simulink model "Simple_4Quad_payload_09_2017a"  (R2018b)
settings: Solver=ode45  StartTime=0.0  StopTime=40  RelTol=1e-3
InitFcn:
  | Simple_4Quad_payload_09_const
values from neighbouring files (symbols this model uses):
  All_rho = [d1 0 0 ... (first row only)    [Colab_4Quad_model_01_const.m]    (also in Colab_4Quad_model_02_const.m; Simple_4Quad_payload_04_const.m; Simple_4Quad_payload_05_const.m; Simple_4Quad_payload_06_const.m)
  alpha_chatt = 0.1    [Simple_4Quad_payload_09_const.m]    (also in Simple_4Quad_payload_10_const.m = 0.001; Simple_4Quad_payload_11_const.m = 0.01; Simple_4Quad_payload_12_const.m = 0.01)
  alphaTF = 0.1    [Simple_4Quad_payload_08_const.m]    (also in Simple_4Quad_payload_09_const.m = 0.5; Simple_4Quad_payload_10_const.m = 1; Simple_4Quad_payload_11_const.m = 0.5; Simple_4Quad_payload_12_const.m = 10)
  B_ob = [zeros(3);eye(3)]    [Simple_4Quad_payload_04_const.m]    (also in Simple_4Quad_payload_05_const.m; Simple_4Quad_payload_06_const.m; Simple_4Quad_payload_07_const.m; Simple_4Quad_payload_08_const.m)
  BBT_inv = ((B'*B)^(-1))*B'    [Simple_2Quad_payload_03_const.m]    (also in Simple_4Quad_payload_04_const.m = ((BR'*BR)^(-1))*BR'; Simple_4Quad_payload_05_const.m = ((BR'*BR)^(-1))*BR'; Simple_4Quad_payload_06_const.m = ((BR'*BR)^(-1))*BR'; Simple_4Quad_payload_07_const.m = ((BR'*BR)^(-1))*BR')
  BR = 1e0*eye(n)    [Simple_4Quad_payload_04_const.m]    (also in Simple_4Quad_payload_05_const.m; Simple_4Quad_payload_06_const.m; Simple_4Quad_payload_07_const.m; Simple_4Quad_payload_08_const.m)
  C_ob = [eye(3) zeros(3)]    [Simple_4Quad_payload_04_const.m]    (also in Simple_4Quad_payload_05_const.m; Simple_4Quad_payload_06_const.m; Simple_4Quad_payload_07_const.m; Simple_4Quad_payload_08_const.m)
  d1 = 0.25    [Colab_4Quad_model_01_const.m]    (also in Colab_4Quad_model_02_const.m = 0.5; Simple_4Quad_payload_01_const.m = 1; Simple_4Quad_payload_02_const.m = 1; Simple_4Quad_payload_03_const.m = 1)
  d2 = 0.25    [Colab_4Quad_model_01_const.m]    (also in Colab_4Quad_model_02_const.m = 0.5; Simple_4Quad_payload_01_const.m = 1; Simple_4Quad_payload_02_const.m = 1; Simple_4Quad_payload_03_const.m = 1)
  Des_rel_dist = 2    [Simple_4Quad_payload_01_const.m]    (also in Simple_4Quad_payload_02_const.m = 4; Simple_4Quad_payload_03_const.m = 4; Simple_4Quad_payload_04_const.m; Simple_4Quad_payload_05_const.m)
  g = 9.81    [Colab_4Quad_model_01_const.m]    (also in Colab_4Quad_model_02_const.m; Simple_2Quad_payload_01_const.m; Simple_2Quad_payload_02_const.m; Simple_2Quad_payload_03_const.m)
  gamma_0 = 1e-0*diag([1e-3;1e-0])    [Simple_2Quad_payload_03_const.m]    (also in Simple_4Quad_payload_04_const.m = 1e-0*diag([1e-6*ones(3,1);1e-0*ones(3,1)]); Simple_4Quad_payload_05_const.m = 1e-1*diag([1e-6*ones(3,1);1e-0*ones(3,1)]); Simple_4Quad_payload_06_const.m = 1e-0*diag([1e-6*ones(3,1);1e-0*ones(3,1)]); Simple_4Quad_payload_07_const.m = 1e-0*diag([1e-6*ones(3,1);1e-0*ones(3,1)]))
  gamma_0L = 1e-0*diag([1e-6*ones(3,1);1e-0*ones(3,1)])    [Simple_4Quad_payload_08_const.m]    (also in Simple_4Quad_payload_09_const.m; Simple_4Quad_payload_10_const.m = 1e+0*diag([1e-3*ones(3,1);1e-3*ones(3,1)]); Simple_4Quad_payload_11_const.m = 1e+0*diag([1e-3*ones(3,1);1e-3*ones(3,1)]); Simple_4Quad_payload_12_const.m = 1e+2*diag(1e-4*ones(3,1)))
  gamma_0v = 1e-0*diag([1e-0*ones(3,1);1e-0*ones(3,1)])    [Simple_4Quad_payload_08_const.m]    (also in Simple_4Quad_payload_09_const.m = 1e-0*diag([1e-6*ones(3,1);1e-6*ones(3,1)]); Simple_4Quad_payload_10_const.m = 1e+0*diag(1e-0*ones(3,1)); Simple_4Quad_payload_11_const.m = 1e+0*diag(1e-0*ones(3,1)); Simple_4Quad_payload_12_const.m = 1e+3*diag(1e-0*ones(3,1)))
  gamma_1 = 1e+2*diag([1e-3;1e-0])    [Simple_2Quad_payload_03_const.m]    (also in Simple_4Quad_payload_04_const.m = 1e+2*diag([1e-6*ones(3,1);1e-0*ones(3,1)]); Simple_4Quad_payload_05_const.m = 1e+2*diag([1e-6*ones(3,1);1e-0*ones(3,1)]); Simple_4Quad_payload_06_const.m = 1e+3*diag([1e-6*ones(3,1);1e-0*ones(3,1)]); Simple_4Quad_payload_07_const.m = 1e+3*diag([1e-6*ones(3,1);1e-0*ones(3,1)]))
  gamma_1L = 1e+3*diag([1e-6*ones(3,1);1e-0*ones(3,1)])    [Simple_4Quad_payload_08_const.m]    (also in Simple_4Quad_payload_09_const.m = 1e+2*diag([1e-6*ones(3,1);1e-0*ones(3,1)]); Simple_4Quad_payload_10_const.m = 1e+1*diag([1e-3*ones(3,1);1e-3*ones(3,1)]); Simple_4Quad_payload_11_const.m = 1e+0*diag([1e-3*ones(3,1);1e-3*ones(3,1)]); Simple_4Quad_payload_12_const.m = 1e+2*diag(1e-4*ones(3,1)))
  gamma_1v = 1e+3*diag([1e-0*ones(3,1);1e-0*ones(3,1)])    [Simple_4Quad_payload_08_const.m]    (also in Simple_4Quad_payload_09_const.m = 1e+2*diag([1e-6*ones(3,1);1e-6*ones(3,1)]); Simple_4Quad_payload_10_const.m = 1e+0*diag(1e-0*ones(3,1)); Simple_4Quad_payload_11_const.m = 1e+0*diag(1e-0*ones(3,1)); Simple_4Quad_payload_12_const.m = 1e+3*diag(1e-0*ones(3,1)))
  Ix = 0.166667    [Colab_4Quad_model_01_const.m]    (also in Colab_4Quad_model_02_const.m = 0.02; Simple_4Quad_payload_01_const.m = 1; Simple_4Quad_payload_02_const.m = 1; Simple_4Quad_payload_03_const.m = 1)
  Iy = 0.166667    [Colab_4Quad_model_01_const.m]    (also in Colab_4Quad_model_02_const.m = 0.02; Simple_4Quad_payload_01_const.m = 1; Simple_4Quad_payload_02_const.m = 1; Simple_4Quad_payload_03_const.m = 1)
  Iz = 0.166667    [Colab_4Quad_model_01_const.m]    (also in Colab_4Quad_model_02_const.m = 0.02; Simple_4Quad_payload_01_const.m = 1; Simple_4Quad_payload_02_const.m = 1; Simple_4Quad_payload_03_const.m = 1)
  Jo = diag([Ix;Iy;Iz])    [Colab_4Quad_model_01_const.m]    (also in Colab_4Quad_model_02_const.m; Simple_4Quad_payload_04_const.m; Simple_4Quad_payload_05_const.m; Simple_4Quad_payload_06_const.m)
  Jq = diag([0.0291 0.0291 0.0552])    [Colab_4Quad_model_01_const.m]    (also in Colab_4Quad_model_02_const.m = diag([0.03 0.03 0.06]); Simple_4Quad_payload_03_const.m = 1.2416e-3 * diag([1 1 2]); Simple_4Quad_payload_04_const.m = 1 * diag([1 1 2]); Simple_4Quad_payload_05_const.m = 1 * diag([1 1 2]))
  k1 = 1    [Simple_2Quad_payload_03_const.m]    (also in Simple_4Quad_payload_04_const.m; Simple_4Quad_payload_05_const.m; Simple_4Quad_payload_06_const.m; Simple_4Quad_payload_07_const.m)
  k2 = 0.1    [Simple_2Quad_payload_03_const.m]    (also in Simple_4Quad_payload_04_const.m; Simple_4Quad_payload_05_const.m; Simple_4Quad_payload_06_const.m; Simple_4Quad_payload_07_const.m)
  l = 3.1819    [Colab_4Quad_model_01_const.m]    (also in Colab_4Quad_model_02_const.m = 3; Simple_2Quad_payload_04_const.m = 1; Simple_4Quad_payload_01_const.m = 1; Simple_4Quad_payload_02_const.m = 2)
  m = 1.5    [Colab_4Quad_model_01_const.m]    (also in Colab_4Quad_model_02_const.m; Simple_2Quad_payload_04_const.m = 1; Simple_4Quad_payload_01_const.m = 1; Simple_4Quad_payload_02_const.m = 1)
  M = 1.0    (= 1)    [Colab_4Quad_model_01_const.m]    (also in Colab_4Quad_model_02_const.m; Simple_2Quad_payload_01_const.m; Simple_2Quad_payload_02_const.m; Simple_2Quad_payload_03_const.m)
  n = 2    [Simple_2Quad_payload_03_const.m]    (also in Simple_4Quad_payload_03_const.m = 6; Simple_4Quad_payload_04_const.m = 6; Simple_4Quad_payload_05_const.m = 6; Simple_4Quad_payload_06_const.m = 6)
  noise_var_Omegao = 0e-6    (= 0)    [Simple_4Quad_payload_07_const.m]    (also in Simple_4Quad_payload_08_const.m; Simple_4Quad_payload_09_const.m; Simple_4Quad_payload_10_const.m; Simple_4Quad_payload_11_const.m)
  noise_var_RelAcc = 0e-6    (= 0)    [Simple_4Quad_payload_07_const.m]    (also in Simple_4Quad_payload_08_const.m; Simple_4Quad_payload_09_const.m; Simple_4Quad_payload_10_const.m; Simple_4Quad_payload_11_const.m)
  noise_var_RelPos = 0e-6    (= 0)    [Simple_4Quad_payload_07_const.m]    (also in Simple_4Quad_payload_08_const.m; Simple_4Quad_payload_09_const.m; Simple_4Quad_payload_10_const.m; Simple_4Quad_payload_11_const.m)
  Q_ob = var_u_ob * eye(6)    [Simple_4Quad_payload_04_const.m]    (also in Simple_4Quad_payload_05_const.m; Simple_4Quad_payload_06_const.m; Simple_4Quad_payload_07_const.m; Simple_4Quad_payload_08_const.m)
  QL = 1e-0*eye(n)    [Simple_4Quad_payload_08_const.m]    (also in Simple_4Quad_payload_09_const.m; Simple_4Quad_payload_10_const.m; Simple_4Quad_payload_11_const.m = 1e-2*eye(n); Simple_4Quad_payload_12_const.m = 1e-0*eye(np))
  QR = 1e-0*eye(n)    [Simple_4Quad_payload_04_const.m]    (also in Simple_4Quad_payload_05_const.m = 1e-1*eye(n); Simple_4Quad_payload_06_const.m; Simple_4Quad_payload_07_const.m; Simple_4Quad_payload_08_const.m)
  Qv = 1e-0*eye(n)    [Simple_4Quad_payload_08_const.m]    (also in Simple_4Quad_payload_09_const.m; Simple_4Quad_payload_10_const.m = 1e-0*eye(np); Simple_4Quad_payload_11_const.m = 1e-2*eye(np); Simple_4Quad_payload_12_const.m = 1e-0*eye(np))
  R = 1e+0*eye(n)    [Simple_2Quad_payload_03_const.m]    (also in Simple_4Quad_payload_04_const.m = 1e+0*eye(m); Simple_4Quad_payload_05_const.m = 1e+0*eye(m); Simple_4Quad_payload_06_const.m; Simple_4Quad_payload_07_const.m)
  R_ob = var_y_ob * eye(3)    [Simple_4Quad_payload_04_const.m]    (also in Simple_4Quad_payload_05_const.m; Simple_4Quad_payload_06_const.m; Simple_4Quad_payload_07_const.m; Simple_4Quad_payload_08_const.m)
  rho_0 = 1e-0    (= 1)    [Simple_2Quad_payload_03_const.m]    (also in Simple_4Quad_payload_04_const.m; Simple_4Quad_payload_05_const.m = 0.1; Simple_4Quad_payload_06_const.m; Simple_4Quad_payload_07_const.m)
  rho_0L = 1e-0    (= 1)    [Simple_4Quad_payload_08_const.m]    (also in Simple_4Quad_payload_09_const.m; Simple_4Quad_payload_10_const.m; Simple_4Quad_payload_11_const.m; Simple_4Quad_payload_12_const.m)
  rho_0v = 1e-1    (= 0.1)    [Simple_4Quad_payload_08_const.m]    (also in Simple_4Quad_payload_09_const.m = 1; Simple_4Quad_payload_10_const.m = 1; Simple_4Quad_payload_11_const.m = 1; Simple_4Quad_payload_12_const.m = 1)
  rho_1 = 1e-0    (= 1)    [Simple_2Quad_payload_03_const.m]    (also in Simple_4Quad_payload_04_const.m; Simple_4Quad_payload_05_const.m; Simple_4Quad_payload_06_const.m; Simple_4Quad_payload_07_const.m)
  rho_1L = 1e-0    (= 1)    [Simple_4Quad_payload_08_const.m]    (also in Simple_4Quad_payload_09_const.m; Simple_4Quad_payload_10_const.m; Simple_4Quad_payload_11_const.m; Simple_4Quad_payload_12_const.m)
  rho_1v = 1e-0    (= 1)    [Simple_4Quad_payload_08_const.m]    (also in Simple_4Quad_payload_09_const.m; Simple_4Quad_payload_10_const.m; Simple_4Quad_payload_11_const.m; Simple_4Quad_payload_12_const.m)
libraries: simulink x1
(part 4 of 4)

== matlab function Simple_4Quad_payload_09_2017a/Controllers and Observers/Controller and Observer - Agent2/Rotational #2/output definition ==
  data: u input; ur output
function ur = fcn(u)

ur = u(4:6);

end

== matlab function Simple_4Quad_payload_09_2017a/Controllers and Observers/Cotnroller and Observer - Agent1 /Rotational #1/CARE ==
  data: P input; a_hat input; BR parameter; R parameter; DP output; QR parameter
function DP = fcn(P,a_hat,BR,R,QR)

DP = a_hat*P + P*a_hat' - P*BR*R*BR'*P + 2*QR;

end

== matlab function Simple_4Quad_payload_09_2017a/Controllers and Observers/Controlelr and Observer - Agent3/Rotational #3/output definition ==
  data: u input; ur output
function ur = fcn(u)

ur = u(4:6);

end

== matlab function Simple_4Quad_payload_09_2017a/Controllers and Observers/Controller and Observer - Agent4/Rotational #4/output definition ==
  data: u input; ur output
function ur = fcn(u)

ur = u(4:6);

end

== matlab function Simple_4Quad_payload_09_2017a/Dynamic model of the entire system/Control inputs from Q1/Controller Interpreter #1 ==
  data: UTi input; qi input; PHIi input; Ui_local_paral output; PHIo input; Ui_local_perpn output
function [Ui_local_paral,Ui_local_perpn] = fcn(UTi,qi,PHIi,PHIo)

phi_i = PHIi(1);
theta_i = PHIi(2);
psi_i = PHIi(3);

Ri = [cos(psi_i)*cos(theta_i) cos(psi_i)*sin(theta_i)*sin(phi_i)-sin(psi_i)*cos(phi_i) cos(psi_i)*sin(theta_i)*cos(phi_i)+sin(psi_i)*sin(phi_i);
    sin(psi_i)*cos(theta_i) sin(psi_i)*sin(theta_i)*sin(phi_i)+cos(psi_i)*cos(phi_i) sin(psi_i)*sin(theta_i)*cos(phi_i)-cos(psi_i)*sin(phi_i);
    -sin(theta_i) cos(theta_i)*sin(phi_i) cos(theta_i)*cos(phi_i)]; 

phio = PHIo(1);
thetao = PHIo(2);
psio = PHIo(3);

Ro = [cos(psio)*cos(thetao) cos(psio)*sin(thetao)*sin(phio)-sin(psio)*cos(phio) cos(psio)*sin(thetao)*cos(phio)+sin(psio)*sin(phio);
    sin(psio)*cos(thetao) sin(psio)*sin(thetao)*sin(phio)+cos(psio)*cos(phio) sin(psio)*sin(thetao)*cos(phio)-cos(psio)*sin(phio);
    -sin(thetao) cos(thetao)*sin(phio) cos(thetao)*cos(phio)];

Ui_local_paral = (qi*qi') * (eye(3) * Ri * UTi); %Ro'
Ui_local_perpn = (eye(3) - qi*qi') * (eye(3) * Ri * UTi); %Ro'


end

== matlab function Simple_4Quad_payload_09_2017a/Controllers and Observers/Cotnroller and Observer - Agent1 /Link #1/CARE ==
  data: P input; a_hat input; BR parameter; R parameter; DP output; QL parameter
function DP = fcn(P,a_hat,BR,R,QL)

DP = a_hat*P + P*a_hat' - P*BR*R*BR'*P + 2*QL;

end

== matlab function Simple_4Quad_payload_09_2017a/Controllers and Observers/Cotnroller and Observer - Agent1 /Link #1/Differentiator/Sliding differentiator ==
  data: u output; u1 input; e input; n parameter; k1 parameter; alpha_chatt parameter
function u = fcn(u1,e,n,k1,alpha_chatt)

b=k1;

ABS = zeros(n,1);
for i=1:n
    if e(i)>0
        ABS(i) = e(i);
    else
        ABS(i) = -e(i);
    end
end
SGN = e ./ (ABS + alpha_chatt);

u = u1 - b*(ABS.^0.5).*SGN;

end

== matlab function Simple_4Quad_payload_09_2017a/Controllers and Observers/Cotnroller and Observer - Agent1 /Link #1/Differentiator/Sliding differentiator1 ==
  data: Du1 output; e input; n parameter; k2 parameter; alpha_chatt parameter
function Du1 = fcn(e,n,k2,alpha_chatt)

a=k2;

ABS = zeros(n,1);
for i=1:n
    if e(i)>0
        ABS(i) = e(i);
    else
        ABS(i) = -e(i);
    end
end
SGN = e ./ (ABS + alpha_chatt);

Du1 = - a*SGN;

end

== matlab function Simple_4Quad_payload_09_2017a/Dynamic model of the entire system/Control inputs from Q2/Controller Interpreter #2 ==
  data: UTi input; qi input; PHIi input; Ui_local_paral output; PHIo input; Ui_local_perpn output
function [Ui_local_paral,Ui_local_perpn] = fcn(UTi,qi,PHIi,PHIo)

phi_i = PHIi(1);
theta_i = PHIi(2);
psi_i = PHIi(3);

Ri = [cos(psi_i)*cos(theta_i) cos(psi_i)*sin(theta_i)*sin(phi_i)-sin(psi_i)*cos(phi_i) cos(psi_i)*sin(theta_i)*cos(phi_i)+sin(psi_i)*sin(phi_i);
    sin(psi_i)*cos(theta_i) sin(psi_i)*sin(theta_i)*sin(phi_i)+cos(psi_i)*cos(phi_i) sin(psi_i)*sin(theta_i)*cos(phi_i)-cos(psi_i)*sin(phi_i);
    -sin(theta_i) cos(theta_i)*sin(phi_i) cos(theta_i)*cos(phi_i)]; 

phio = PHIo(1);
thetao = PHIo(2);
psio = PHIo(3);

Ro = [cos(psio)*cos(thetao) cos(psio)*sin(thetao)*sin(phio)-sin(psio)*cos(phio) cos(psio)*sin(thetao)*cos(phio)+sin(psio)*sin(phio);
    sin(psio)*cos(thetao) sin(psio)*sin(thetao)*sin(phio)+cos(psio)*cos(phio) sin(psio)*sin(thetao)*cos(phio)-cos(psio)*sin(phio);
    -sin(thetao) cos(thetao)*sin(phio) cos(thetao)*cos(phio)];

Ui_local_paral = (qi*qi') * (eye(3) * Ri * UTi); %Ro'
Ui_local_perpn = (eye(3) - qi*qi') * (eye(3) * Ri * UTi); %Ro'


end

== matlab function Simple_4Quad_payload_09_2017a/Dynamic model of the entire system/Control inputs from Q3/Controller Interpreter #3 ==
  data: UTi input; qi input; PHIi input; Ui_local_paral output; PHIo input; Ui_local_perpn output
function [Ui_local_paral,Ui_local_perpn] = fcn(UTi,qi,PHIi,PHIo)

phi_i = PHIi(1);
theta_i = PHIi(2);
psi_i = PHIi(3);

Ri = [cos(psi_i)*cos(theta_i) cos(psi_i)*sin(theta_i)*sin(phi_i)-sin(psi_i)*cos(phi_i) cos(psi_i)*sin(theta_i)*cos(phi_i)+sin(psi_i)*sin(phi_i);
    sin(psi_i)*cos(theta_i) sin(psi_i)*sin(theta_i)*sin(phi_i)+cos(psi_i)*cos(phi_i) sin(psi_i)*sin(theta_i)*cos(phi_i)-cos(psi_i)*sin(phi_i);
    -sin(theta_i) cos(theta_i)*sin(phi_i) cos(theta_i)*cos(phi_i)]; 

phio = PHIo(1);
thetao = PHIo(2);
psio = PHIo(3);

Ro = [cos(psio)*cos(thetao) cos(psio)*sin(thetao)*sin(phio)-sin(psio)*cos(phio) cos(psio)*sin(thetao)*cos(phio)+sin(psio)*sin(phio);
    sin(psio)*cos(thetao) sin(psio)*sin(thetao)*sin(phio)+cos(psio)*cos(phio) sin(psio)*sin(thetao)*cos(phio)-cos(psio)*sin(phio);
    -sin(thetao) cos(thetao)*sin(phio) cos(thetao)*cos(phio)];

Ui_local_paral = (qi*qi') * (eye(3) * Ri * UTi); %Ro'
Ui_local_perpn = (eye(3) - qi*qi') * (eye(3) * Ri * UTi); %Ro'


end

== matlab function Simple_4Quad_payload_09_2017a/Dynamic model of the entire system/Control inputs from Q4/Controller Interpreter #4 ==
  data: UTi input; qi input; PHIi input; Ui_local_paral output; PHIo input; Ui_local_perpn output
function [Ui_local_paral,Ui_local_perpn] = fcn(UTi,qi,PHIi,PHIo)

phi_i = PHIi(1);
theta_i = PHIi(2);
psi_i = PHIi(3);

Ri = [cos(psi_i)*cos(theta_i) cos(psi_i)*sin(theta_i)*sin(phi_i)-sin(psi_i)*cos(phi_i) cos(psi_i)*sin(theta_i)*cos(phi_i)+sin(psi_i)*sin(phi_i);
    sin(psi_i)*cos(theta_i) sin(psi_i)*sin(theta_i)*sin(phi_i)+cos(psi_i)*cos(phi_i) sin(psi_i)*sin(theta_i)*cos(phi_i)-cos(psi_i)*sin(phi_i);
    -sin(theta_i) cos(theta_i)*sin(phi_i) cos(theta_i)*cos(phi_i)]; 

phio = PHIo(1);
thetao = PHIo(2);
psio = PHIo(3);

Ro = [cos(psio)*cos(thetao) cos(psio)*sin(thetao)*sin(phio)-sin(psio)*cos(phio) cos(psio)*sin(thetao)*cos(phio)+sin(psio)*sin(phio);
    sin(psio)*cos(thetao) sin(psio)*sin(thetao)*sin(phio)+cos(psio)*cos(phio) sin(psio)*sin(thetao)*cos(phio)-cos(psio)*sin(phio);
    -sin(thetao) cos(thetao)*sin(phio) cos(thetao)*cos(phio)];

Ui_local_paral = (qi*qi') * (eye(3) * Ri * UTi); %Ro'
Ui_local_perpn = (eye(3) - qi*qi') * (eye(3) * Ri * UTi); %Ro'


end

== matlab function Simple_4Quad_payload_09_2017a/Controllers and Observers/Cotnroller and Observer - Agent1 /Link #1/g-Estimator ==
  data: sigma input; g_hat input; P input; rho_1L parameter; gamma_1L parameter; Dg_hat output
function Dg_hat = fcn(sigma,g_hat,P,rho_1L,gamma_1L)

Dg_hat = - gamma_1L * P * sigma - rho_1L * gamma_1L * g_hat;

end

== matlab function Simple_4Quad_payload_09_2017a/Controllers and Observers/Cotnroller and Observer - Agent1 /Link #1/g-Estimator1 ==
  data: sigma input; x input; P input; rho_0L parameter; gamma_0L parameter; Da_hat output; a_hat input
function Da_hat = fcn(sigma,x,P,rho_0L,gamma_0L,a_hat)

DVa_hat = - gamma_0L * P * diag(sigma) * (x - sigma) - rho_0L * gamma_0L * diag(a_hat);

Da_hat = diag(DVa_hat);

end

== matlab function Simple_4Quad_payload_09_2017a/Controllers and Observers/Cotnroller and Observer - Agent1 /Link #1/main ==
  data: sigma input; zeta input; u output; Dy_d input; R parameter; P input; a_hat input; BR parameter; g_hat input; x input; QL parameter; BBT_inv parameter; n parameter
function u = fcn(sigma,zeta,Dy_d,R,P,a_hat,BR,g_hat,x,QL,BBT_inv,n)

u1 = (1/2) * R * BR' * P * sigma;
u2 = BBT_inv * (Dy_d - a_hat*x + (eye(n) + 2*(((P)^(-1)*QL)) + a_hat)*sigma - g_hat - zeta) - (3/4) * R * BR' * P * sigma;

u = u1 + u2;

end

== matlab function Simple_4Quad_payload_09_2017a/Controllers and Observers/Cotnroller and Observer - Agent1 /Link #1/output definition ==
  data: u input; ur output
function ur = fcn(u)

ur = u(4:6);

end

== matlab function Simple_4Quad_payload_09_2017a/Controllers and Observers/Cotnroller and Observer - Agent1 /Link #1/variable change ==
  data: X input; Xd input; x_mod output; u input; xd_mod output; e_mod output
function [x_mod,xd_mod,e_mod] = fcn(X,Xd,u)

x_mod = X;

xd_mod = [Xd;u(1:3)];

e_mod = xd_mod - x_mod;


end

== matlab function Simple_4Quad_payload_09_2017a/Controllers and Observers/Controller and Observer - Agent2/Link #2/CARE ==
  data: P input; a_hat input; BR parameter; R parameter; DP output; QL parameter
function DP = fcn(P,a_hat,BR,R,QL)

DP = a_hat*P + P*a_hat' - P*BR*R*BR'*P + 2*QL;

end

== matlab function Simple_4Quad_payload_09_2017a/Controllers and Observers/Controller and Observer - Agent2/Link #2/Differentiator/Sliding differentiator ==
  data: u output; u1 input; e input; n parameter; k1 parameter; alpha_chatt parameter
function u = fcn(u1,e,n,k1,alpha_chatt)

b=k1;

ABS = zeros(n,1);
for i=1:n
    if e(i)>0
        ABS(i) = e(i);
    else
        ABS(i) = -e(i);
    end
end
SGN = e ./ (ABS + alpha_chatt);

u = u1 - b*(ABS.^0.5).*SGN;

end

== matlab function Simple_4Quad_payload_09_2017a/Controllers and Observers/Controller and Observer - Agent2/Link #2/Differentiator/Sliding differentiator1 ==
  data: Du1 output; e input; n parameter; k2 parameter; alpha_chatt parameter
function Du1 = fcn(e,n,k2,alpha_chatt)

a=k2;

ABS = zeros(n,1);
for i=1:n
    if e(i)>0
        ABS(i) = e(i);
    else
        ABS(i) = -e(i);
    end
end
SGN = e ./ (ABS + alpha_chatt);

Du1 = - a*SGN;

end

== matlab function Simple_4Quad_payload_09_2017a/Controllers and Observers/Controller and Observer - Agent2/Link #2/g-Estimator ==
  data: sigma input; g_hat input; P input; rho_1L parameter; gamma_1L parameter; Dg_hat output
function Dg_hat = fcn(sigma,g_hat,P,rho_1L,gamma_1L)

Dg_hat = - gamma_1L * P * sigma - rho_1L * gamma_1L * g_hat;

end

== matlab function Simple_4Quad_payload_09_2017a/Controllers and Observers/Controller and Observer - Agent2/Link #2/g-Estimator1 ==
  data: sigma input; x input; P input; rho_0L parameter; gamma_0L parameter; Da_hat output; a_hat input
function Da_hat = fcn(sigma,x,P,rho_0L,gamma_0L,a_hat)

DVa_hat = - gamma_0L * P * diag(sigma) * (x - sigma) - rho_0L * gamma_0L * diag(a_hat);

Da_hat = diag(DVa_hat);

end

== matlab function Simple_4Quad_payload_09_2017a/Controllers and Observers/Controller and Observer - Agent2/Link #2/main ==
  data: sigma input; zeta input; u output; Dy_d input; R parameter; P input; a_hat input; BR parameter; g_hat input; x input; QL parameter; BBT_inv parameter; n parameter
function u = fcn(sigma,zeta,Dy_d,R,P,a_hat,BR,g_hat,x,QL,BBT_inv,n)

u1 = (1/2) * R * BR' * P * sigma;
u2 = BBT_inv * (Dy_d - a_hat*x + (eye(n) + 2*(((P)^(-1)*QL)) + a_hat)*sigma - g_hat - zeta) - (3/4) * R * BR' * P * sigma;

u = u1 + u2;

end

== matlab function Simple_4Quad_payload_09_2017a/Controllers and Observers/Controller and Observer - Agent2/Link #2/output definition ==
  data: u input; ur output
function ur = fcn(u)

ur = u(4:6);

end

== matlab function Simple_4Quad_payload_09_2017a/Controllers and Observers/Controller and Observer - Agent2/Link #2/variable change ==
  data: X input; Xd input; x_mod output; u input; xd_mod output; e_mod output
function [x_mod,xd_mod,e_mod] = fcn(X,Xd,u)

x_mod = X;

xd_mod = [Xd;u(1:3)];

e_mod = xd_mod - x_mod;


end

== matlab function Simple_4Quad_payload_09_2017a/Controllers and Observers/Controlelr and Observer - Agent3/Link #3/CARE ==
  data: P input; a_hat input; BR parameter; R parameter; DP output; QL parameter
function DP = fcn(P,a_hat,BR,R,QL)

DP = a_hat*P + P*a_hat' - P*BR*R*BR'*P + 2*QL;

end

== matlab function Simple_4Quad_payload_09_2017a/Controllers and Observers/Controlelr and Observer - Agent3/Link #3/Differentiator/Sliding differentiator ==
  data: u output; u1 input; e input; n parameter; k1 parameter; alpha_chatt parameter
function u = fcn(u1,e,n,k1,alpha_chatt)

b=k1;

ABS = zeros(n,1);
for i=1:n
    if e(i)>0
        ABS(i) = e(i);
    else
        ABS(i) = -e(i);
    end
end
SGN = e ./ (ABS + alpha_chatt);

u = u1 - b*(ABS.^0.5).*SGN;

end

== matlab function Simple_4Quad_payload_09_2017a/Controllers and Observers/Cotnroller and Observer - Agent1 /Rotational #1/Differentiator/Sliding differentiator ==
  data: u output; u1 input; e input; n parameter; k1 parameter; alpha_chatt parameter
function u = fcn(u1,e,n,k1,alpha_chatt)

b=k1;

ABS = zeros(n,1);
for i=1:n
    if e(i)>0
        ABS(i) = e(i);
    else
        ABS(i) = -e(i);
    end
end
SGN = e ./ (ABS + alpha_chatt);

u = u1 - b*(ABS.^0.5).*SGN;

end

== matlab function Simple_4Quad_payload_09_2017a/Controllers and Observers/Controlelr and Observer - Agent3/Link #3/Differentiator/Sliding differentiator1 ==
  data: Du1 output; e input; n parameter; k2 parameter; alpha_chatt parameter
function Du1 = fcn(e,n,k2,alpha_chatt)

a=k2;

ABS = zeros(n,1);
for i=1:n
    if e(i)>0
        ABS(i) = e(i);
    else
        ABS(i) = -e(i);
    end
end
SGN = e ./ (ABS + alpha_chatt);

Du1 = - a*SGN;

end

== matlab function Simple_4Quad_payload_09_2017a/Controllers and Observers/Controlelr and Observer - Agent3/Link #3/g-Estimator ==
  data: sigma input; g_hat input; P input; rho_1L parameter; gamma_1L parameter; Dg_hat output
function Dg_hat = fcn(sigma,g_hat,P,rho_1L,gamma_1L)

Dg_hat = - gamma_1L * P * sigma - rho_1L * gamma_1L * g_hat;

end

== matlab function Simple_4Quad_payload_09_2017a/Controllers and Observers/Controlelr and Observer - Agent3/Link #3/g-Estimator1 ==
  data: sigma input; x input; P input; rho_0L parameter; gamma_0L parameter; Da_hat output; a_hat input
function Da_hat = fcn(sigma,x,P,rho_0L,gamma_0L,a_hat)

DVa_hat = - gamma_0L * P * diag(sigma) * (x - sigma) - rho_0L * gamma_0L * diag(a_hat);

Da_hat = diag(DVa_hat);

end

== matlab function Simple_4Quad_payload_09_2017a/Controllers and Observers/Controlelr and Observer - Agent3/Link #3/main ==
  data: sigma input; zeta input; u output; Dy_d input; R parameter; P input; a_hat input; BR parameter; g_hat input; x input; QL parameter; BBT_inv parameter; n parameter
function u = fcn(sigma,zeta,Dy_d,R,P,a_hat,BR,g_hat,x,QL,BBT_inv,n)

u1 = (1/2) * R * BR' * P * sigma;
u2 = BBT_inv * (Dy_d - a_hat*x + (eye(n) + 2*(((P)^(-1)*QL)) + a_hat)*sigma - g_hat - zeta) - (3/4) * R * BR' * P * sigma;

u = u1 + u2;

end

== matlab function Simple_4Quad_payload_09_2017a/Controllers and Observers/Controlelr and Observer - Agent3/Link #3/output definition ==
  data: u input; ur output
function ur = fcn(u)

ur = u(4:6);

end

== matlab function Simple_4Quad_payload_09_2017a/Controllers and Observers/Controlelr and Observer - Agent3/Link #3/variable change ==
  data: X input; Xd input; x_mod output; u input; xd_mod output; e_mod output
function [x_mod,xd_mod,e_mod] = fcn(X,Xd,u)

x_mod = X;

xd_mod = [Xd;u(1:3)];

e_mod = xd_mod - x_mod;


end

== matlab function Simple_4Quad_payload_09_2017a/Controllers and Observers/Cotnroller and Observer - Agent1 /Controller Interpreter #1 ==
  data: Trust1 output; ut_1 input; PHI_d_1 output
function [Trust1,PHI_d_1] = fcn(ut_1)

%%
fT_1 = sqrt((ut_1(1)^2)+(ut_1(2)^2)+(ut_1(3)^2));
psi_d_1 = 0;
phi_d_1 = asin( min(max(((sin(psi_d_1)*ut_1(1) - cos(psi_d_1)*ut_1(2)) / (fT_1+1e-3)),-1),1) );
theta_d_1 = atan( (cos(psi_d_1)*ut_1(1) + sin(psi_d_1)*ut_1(2)) / (ut_1(3)+1e-3) );
PHI_d_1 = [phi_d_1;theta_d_1;psi_d_1]; 
Trust1 = [0;0;fT_1];

end

== matlab function Simple_4Quad_payload_09_2017a/Controllers and Observers/Cotnroller and Observer - Agent1 /Rotational #1/Differentiator/Sliding differentiator1 ==
  data: Du1 output; e input; n parameter; k2 parameter; alpha_chatt parameter
function Du1 = fcn(e,n,k2,alpha_chatt)

a=k2;

ABS = zeros(n,1);
for i=1:n
    if e(i)>0
        ABS(i) = e(i);
    else
        ABS(i) = -e(i);
    end
end
SGN = e ./ (ABS + alpha_chatt);

Du1 = - a*SGN;

end

== matlab function Simple_4Quad_payload_09_2017a/Controllers and Observers/Cotnroller and Observer - Agent1 /Rotational #1/g-Estimator ==
  data: sigma input; g_hat input; P input; rho_1 parameter; gamma_1 parameter; Dg_hat output
function Dg_hat = fcn(sigma,g_hat,P,rho_1,gamma_1)

Dg_hat = - gamma_1 * P * sigma - rho_1 * gamma_1 * g_hat;

end

== matlab function Simple_4Quad_payload_09_2017a/Controllers and Observers/Cotnroller and Observer - Agent1 /Rotational #1/g-Estimator1 ==
  data: sigma input; x input; P input; rho_0 parameter; gamma_0 parameter; Da_hat output; a_hat input
function Da_hat = fcn(sigma,x,P,rho_0,gamma_0,a_hat)

DVa_hat = - gamma_0 * P * diag(sigma) * (x - sigma) - rho_0 * gamma_0 * diag(a_hat);

Da_hat = diag(DVa_hat);

end

== matlab function Simple_4Quad_payload_09_2017a/Controllers and Observers/Cotnroller and Observer - Agent1 /Rotational #1/main ==
  data: sigma input; zeta input; u output; Dy_d input; R parameter; P input; a_hat input; BR parameter; g_hat input; x input; QR parameter; BBT_inv parameter; n parameter
function u = fcn(sigma,zeta,Dy_d,R,P,a_hat,BR,g_hat,x,QR,BBT_inv,n)

u1 = (1/2) * R * BR' * P * sigma;
u2 = BBT_inv * (Dy_d - a_hat*x + (eye(n) + 2*(((P)^(-1)*QR)) + a_hat)*sigma - g_hat - zeta) - (3/4) * R * BR' * P * sigma;

u = u1 + u2;

end

== matlab function Simple_4Quad_payload_09_2017a/Controllers and Observers/Cotnroller and Observer - Agent1 /Rotational #1/variable change ==
  data: X input; Xd input; x_mod output; u input; xd_mod output; e_mod output
function [x_mod,xd_mod,e_mod] = fcn(X,Xd,u)

x_mod = X;

xd_mod = [Xd;u(1:3)];

e_mod = xd_mod - x_mod;


end

== matlab function Simple_4Quad_payload_09_2017a/Controllers and Observers/Controller and Observer - Agent4/Link #4/CARE ==
  data: P input; a_hat input; BR parameter; R parameter; DP output; QL parameter
function DP = fcn(P,a_hat,BR,R,QL)

DP = a_hat*P + P*a_hat' - P*BR*R*BR'*P + 2*QL;

end

== matlab function Simple_4Quad_payload_09_2017a/Controllers and Observers/Controller and Observer - Agent4/Link #4/Differentiator/Sliding differentiator ==
  data: u output; u1 input; e input; n parameter; k1 parameter; alpha_chatt parameter
function u = fcn(u1,e,n,k1,alpha_chatt)

b=k1;

ABS = zeros(n,1);
for i=1:n
    if e(i)>0
        ABS(i) = e(i);
    else
        ABS(i) = -e(i);
    end
end
SGN = e ./ (ABS + alpha_chatt);

u = u1 - b*(ABS.^0.5).*SGN;

end

== matlab function Simple_4Quad_payload_09_2017a/Controllers and Observers/Controller and Observer - Agent4/Link #4/Differentiator/Sliding differentiator1 ==
  data: Du1 output; e input; n parameter; k2 parameter; alpha_chatt parameter
function Du1 = fcn(e,n,k2,alpha_chatt)

a=k2;

ABS = zeros(n,1);
for i=1:n
    if e(i)>0
        ABS(i) = e(i);
    else
        ABS(i) = -e(i);
    end
end
SGN = e ./ (ABS + alpha_chatt);

Du1 = - a*SGN;

end

== matlab function Simple_4Quad_payload_09_2017a/Controllers and Observers/Controller and Observer - Agent4/Link #4/g-Estimator ==
  data: sigma input; g_hat input; P input; rho_1L parameter; gamma_1L parameter; Dg_hat output
function Dg_hat = fcn(sigma,g_hat,P,rho_1L,gamma_1L)

Dg_hat = - gamma_1L * P * sigma - rho_1L * gamma_1L * g_hat;

end

== matlab function Simple_4Quad_payload_09_2017a/Rotational Controller Log/For matrix Plot/MATLAB Function ==
  data: u input; y output
function y = fcn(u)
S1 = size(u,1);
S2 = size(u,2);

y = zeros(S1*S2,1);
num = 0;
for i=1:S1
    for j=1:S2
        num = num + 1;
        y(num,1) = u(i,j);
    end
end

end

== matlab function Simple_4Quad_payload_09_2017a/Rotational Controller Log/For matrix Plot1/MATLAB Function ==
  data: u input; y output
function y = fcn(u)
S1 = size(u,1);
S2 = size(u,2);

y = zeros(S1*S2,1);
num = 0;
for i=1:S1
    for j=1:S2
        num = num + 1;
        y(num,1) = u(i,j);
    end
end

end

== matlab function Simple_4Quad_payload_09_2017a/Rotational Controller Log/For matrix Plot2/MATLAB Function ==
  data: u input; y output
function y = fcn(u)
S1 = size(u,1);
S2 = size(u,2);

y = zeros(S1*S2,1);
num = 0;
for i=1:S1
    for j=1:S2
        num = num + 1;
        y(num,1) = u(i,j);
    end
end

end

== matlab function Simple_4Quad_payload_09_2017a/Rotational Controller Log/For matrix Plot3/MATLAB Function ==
  data: u input; y output
function y = fcn(u)
S1 = size(u,1);
S2 = size(u,2);

y = zeros(S1*S2,1);
num = 0;
for i=1:S1
    for j=1:S2
        num = num + 1;
        y(num,1) = u(i,j);
    end
end

end

== matlab function Simple_4Quad_payload_09_2017a/Rotational Controller Log/For matrix Plot4/MATLAB Function ==
  data: u input; y output
function y = fcn(u)
S1 = size(u,1);
S2 = size(u,2);

y = zeros(S1*S2,1);
num = 0;
for i=1:S1
    for j=1:S2
        num = num + 1;
        y(num,1) = u(i,j);
    end
end

end

== matlab function Simple_4Quad_payload_09_2017a/Rotational Controller Log/For matrix Plot5/MATLAB Function ==
  data: u input; y output
function y = fcn(u)
S1 = size(u,1);
S2 = size(u,2);

y = zeros(S1*S2,1);
num = 0;
for i=1:S1
    for j=1:S2
        num = num + 1;
        y(num,1) = u(i,j);
    end
end

end

== matlab function Simple_4Quad_payload_09_2017a/Controllers and Observers/Controller and Observer - Agent4/Link #4/g-Estimator1 ==
  data: sigma input; x input; P input; rho_0L parameter; gamma_0L parameter; Da_hat output; a_hat input
function Da_hat = fcn(sigma,x,P,rho_0L,gamma_0L,a_hat)

DVa_hat = - gamma_0L * P * diag(sigma) * (x - sigma) - rho_0L * gamma_0L * diag(a_hat);

Da_hat = diag(DVa_hat);

end

== matlab function Simple_4Quad_payload_09_2017a/Controllers and Observers/Controller and Observer - Agent4/Link #4/main ==
  data: sigma input; zeta input; u output; Dy_d input; R parameter; P input; a_hat input; BR parameter; g_hat input; x input; QL parameter; BBT_inv parameter; n parameter
function u = fcn(sigma,zeta,Dy_d,R,P,a_hat,BR,g_hat,x,QL,BBT_inv,n)

u1 = (1/2) * R * BR' * P * sigma;
u2 = BBT_inv * (Dy_d - a_hat*x + (eye(n) + 2*(((P)^(-1)*QL)) + a_hat)*sigma - g_hat - zeta) - (3/4) * R * BR' * P * sigma;

u = u1 + u2;

end

== matlab function Simple_4Quad_payload_09_2017a/Controllers and Observers/Controller and Observer - Agent4/Link #4/output definition ==
  data: u input; ur output
function ur = fcn(u)

ur = u(4:6);

end

== matlab function Simple_4Quad_payload_09_2017a/Controllers and Observers/Controller and Observer - Agent4/Link #4/variable change ==
  data: X input; Xd input; x_mod output; u input; xd_mod output; e_mod output
function [x_mod,xd_mod,e_mod] = fcn(X,Xd,u)

x_mod = X;

xd_mod = [Xd;u(1:3)];

e_mod = xd_mod - x_mod;


end

== matlab function Simple_4Quad_payload_09_2017a/Controllers and Observers/Controller - Payload/Payload/CARE ==
  data: P input; a_hat input; BR parameter; R parameter; DP output; Qv parameter
function DP = fcn(P,a_hat,BR,R,Qv)

DP = a_hat*P + P*a_hat' - P*BR*R*BR'*P + 2*Qv;

end

== matlab function Simple_4Quad_payload_09_2017a/Rotational Controller Log/For matrix Plot6/MATLAB Function ==
  data: u input; y output
function y = fcn(u)
S1 = size(u,1);
S2 = size(u,2);

y = zeros(S1*S2,1);
num = 0;
for i=1:S1
    for j=1:S2
        num = num + 1;
        y(num,1) = u(i,j);
    end
end

end

== matlab function Simple_4Quad_payload_09_2017a/Controllers and Observers/Controller - Payload/Payload/Differentiator/Sliding differentiator ==
  data: u output; u1 input; e input; n parameter; k1 parameter; alpha_chatt parameter
function u = fcn(u1,e,n,k1,alpha_chatt)

b=k1;

ABS = zeros(n,1);
for i=1:n
    if e(i)>0
        ABS(i) = e(i);
    else
        ABS(i) = -e(i);
    end
end
SGN = e ./ (ABS + alpha_chatt);

u = u1 - b*(ABS.^0.5).*SGN;

end

== matlab function Simple_4Quad_payload_09_2017a/Rotational Controller Log/For matrix Plot7/MATLAB Function ==
  data: u input; y output
function y = fcn(u)
S1 = size(u,1);
S2 = size(u,2);

y = zeros(S1*S2,1);
num = 0;
for i=1:S1
    for j=1:S2
        num = num + 1;
        y(num,1) = u(i,j);
    end
end

end

== matlab function Simple_4Quad_payload_09_2017a/Controllers and Observers/Controller - Payload/Payload/Differentiator/Sliding differentiator1 ==
  data: Du1 output; e input; n parameter; k2 parameter; alpha_chatt parameter
function Du1 = fcn(e,n,k2,alpha_chatt)

a=k2;

ABS = zeros(n,1);
for i=1:n
    if e(i)>0
        ABS(i) = e(i);
    else
        ABS(i) = -e(i);
    end
end
SGN = e ./ (ABS + alpha_chatt);

Du1 = - a*SGN;

end

== matlab function Simple_4Quad_payload_09_2017a/Controllers and Observers/Controller - Payload/Payload/g-Estimator ==
  data: sigma input; g_hat input; P input; rho_1v parameter; gamma_1v parameter; Dg_hat output
function Dg_hat = fcn(sigma,g_hat,P,rho_1v,gamma_1v)

Dg_hat = - gamma_1v * P * sigma - rho_1v * gamma_1v * g_hat;

end

== matlab function Simple_4Quad_payload_09_2017a/Controllers and Observers/Controller - Payload/Payload/g-Estimator1 ==
  data: sigma input; x input; P input; rho_0v parameter; gamma_0v parameter; Da_hat output; a_hat input
function Da_hat = fcn(sigma,x,P,rho_0v,gamma_0v,a_hat)

DVa_hat = - gamma_0v * P * diag(sigma) * (x - sigma) - rho_0v * gamma_0v * diag(a_hat);

Da_hat = diag(DVa_hat);

end

== matlab function Simple_4Quad_payload_09_2017a/Controllers and Observers/Controller - Payload/Payload/main ==
  data: sigma input; zeta input; u output; Dy_d input; R parameter; P input; a_hat input; BR parameter; g_hat input; x input; Qv parameter; BBT_inv parameter; n parameter
function u = fcn(sigma,zeta,Dy_d,R,P,a_hat,BR,g_hat,x,Qv,BBT_inv,n)

u1 = (1/2) * R * BR' * P * sigma;
u2 = BBT_inv * (Dy_d - a_hat*x + (eye(n) + 2*(((P)^(-1)*Qv)) + a_hat)*sigma - g_hat - zeta) - (3/4) * R * BR' * P * sigma;

u = u1 + u2;

end

== matlab function Simple_4Quad_payload_09_2017a/Controllers and Observers/Controller - Payload/Payload/variable change ==
  data: X input; Xd input; x_mod output; xd_mod output; e_mod output
function [x_mod,xd_mod,e_mod] = fcn(X,Xd)

x_mod = X;

xd_mod = Xd;

e_mod = xd_mod - x_mod;


end

== matlab function Simple_4Quad_payload_09_2017a/Controllers and Observers/Controller - Payload/Rotation_Q1/D Phi ==
  data: Omega_O input; D_PHI_O output; PHI_O input
function D_PHI_O = fcn(Omega_O,PHI_O)

phi_O = PHI_O(1);
theta_O = PHI_O(2);

Rm_O = [1 0 -sin(theta_O);
    0 cos(phi_O) cos(theta_O)*sin(phi_O);
    0 -sin(phi_O) cos(theta_O)*cos(phi_O)];

D_PHI_O = (Rm_O)^(-1) * Omega_O;


end
